simulink model "test_5ph_core_coupling"  (R2018b)
settings: Solver=VariableStepAuto  StartTime=0.0  StopTime=10.0  RelTol=1e-3
undefined symbols (not defined in the file): Five, Phase
libraries: powerlib x12, typhoonHILlib x1
settings Model: Creator=Marcos  LastModifiedBy=USER
settings SFSimCC: SimUseLocalCustomCode=off
settings RTWCC: RTWUseLocalCustomCode=off

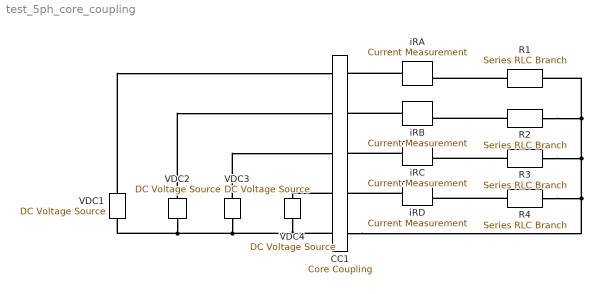
== system test_5ph_core_coupling ==
  CC1 : typhoonHILlib/Core Coupling  CouplingPhases=Five-Phase  IsTLM=off  snb_type_i=None  R1=100e3  C1=1e-6  fixed_snb_i=off  snb_type_v=None  R2=100e3  L1=1e-3  fixed_snb_v=off  CouplingType=Inductive  coup_cap=1e-3  coup_ind=1e-3  toggle_init=on  model_loaded=off  old_pat=typhoonPatterns/5P CC  old_size=15,196
      settings: SourceProductName=Typhoon HIL
  R{1..4} (4 alike) : powerlib/Elements/Series RLC Branch  LConnTagsString=__new0  RConnTagsString=__new0  BranchType=R  Resistance=10  Inductance=1e-3  SetiL0=off  InitialCurrent=0  Capacitance=1e-6  Setx0=off  InitialVoltage=0  Measurements=None
      settings: SourceProductName=Simscape Electrical
  VDC{1..4} (4 alike) : powerlib/Electrical Sources/DC Voltage Source  Amplitude=100  Measurements=None
      settings: SourceProductName=Simscape Electrical
  iRA : powerlib/Measurements/Current Measurement  PhasorSimulation=off  OutputType=Complex  PSBequivalent=0
      settings: SourceProductName=Simscape Electrical
  iRB : powerlib/Measurements/Current Measurement  PhasorSimulation=off  OutputType=Complex  PSBequivalent=0
      settings: SourceProductName=Simscape Electrical
  iRC : powerlib/Measurements/Current Measurement  PhasorSimulation=off  OutputType=Complex  PSBequivalent=0
      settings: SourceProductName=Simscape Electrical
  iRD : powerlib/Measurements/Current Measurement  PhasorSimulation=off  OutputType=Complex  PSBequivalent=0
      settings: SourceProductName=Simscape Electrical
  connections:
  R1/LConn1 -- iRA/RConn1
  iRA/LConn1 -- CC1/RConn1
  R2/LConn1 -- iRB/RConn1
  R3/LConn1 -- iRC/RConn1
  iRB/LConn1 -- CC1/RConn2
  iRC/LConn1 -- CC1/RConn3
  iRD/LConn1 -- CC1/RConn4
  R4/LConn1 -- iRD/RConn1
  CC1/RConn5 -- R4/RConn1 -- R3/RConn1 -- R2/RConn1 -- R1/RConn1
  CC1/LConn5 -- VDC4/LConn1 -- VDC3/LConn1 -- VDC2/LConn1 -- VDC1/LConn1
  VDC1/RConn1 -- CC1/LConn1
  VDC2/RConn1 -- CC1/LConn2
  VDC3/RConn1 -- CC1/LConn3
  CC1/LConn4 -- VDC4/RConn1
